simulink model "sl_subsys_fcncallerr10"  (Simulink 7.6)
settings: Solver=FixedStepDiscrete  StartTime=0.0  StopTime=10.0  FixedStep=1  RelTol=1e-3
Description:
  | Nested data dependency violation
  | 
  | To execute f2() we require that its data input, d be
  | valid. This means f1/Gain must execute before f1/chart2.
  | However, f1/chart2 is driving f1/Gain resulting in
  | a data dependency violation.
settings Model: Creator=The MathWorks Inc.  CovMetricSettings=d  ExtModeAutoUpdateStatusClock=off
settings OptimizationCC: BlockReduction=off  BooleanDataType=off  InlineInvariantSignals=on  InitFltsAndDblsToZero=on
settings DebuggingCC: SaveWithParameterizedLinksMsg=none  SignalResolutionControl=TryResolveAllWithWarning  SolverPrmCheckMsg=none  MultiTaskDSMMsg=warning  MultiTaskCondExecSysMsg=none  UnconnectedInputMsg=none  UnconnectedOutputMsg=none  UnconnectedLineMsg=none
settings HardwareCC: TargetUnknown=on
settings SFSimCC: SimParseCustomCode=off
settings RTWCC: IncludeERTFirstTime=on
settings CodeAppCC: CustomSymbolStrFcn=$F$N$M
settings GRTTargetCC: TargetFcnLib=ansi_tfl_tmw.mat

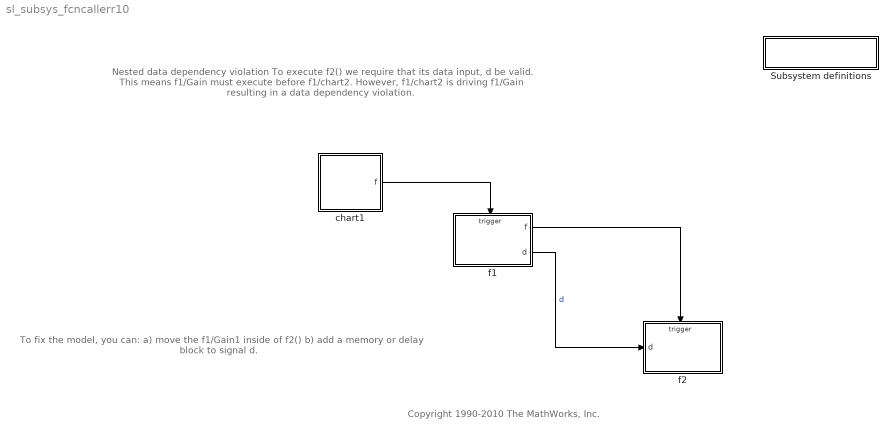
== system sl_subsys_fcncallerr10 ==
  note: Nested data dependency violation
      |
      | To execute f2() we require that its data input, d be
      | valid. This means f1/Gain must execute before f1/chart2.
      | However, f1/chart2 is driving f1/Gain resulting in
      | a data dependency violation.
  note: To fix the model, you can:
      | a)  move the f1/Gain1 inside of f2()
      | b) add a memory or delay block to signal d.
  note: Copyright 1990-2010 The MathWorks, Inc.
  " Subsystem definitions" : Subsystem
      settings: OpenFcn=helpview([matlabroot,'/toolbox/simulink/simdemos/simfeatures/html/sl_subsys_definitions.html']);
      mask Display: disp('Subsystem\ndefinitions')
  chart1 : Stateflow chart  TreatAsAtomicUnit=on
  f1 : Subsystem  TreatAsAtomicUnit=on
  f2 : Subsystem  TreatAsAtomicUnit=on
  wires:
  chart1/1(f) -> f1/Trigger
  f1/1(f) -> f2/Trigger
  f1/2(d) -> f2/1(d)  "d"

== system sl_subsys_fcncallerr10/ Subsystem definitions ==

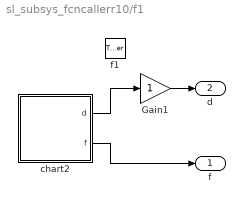
== system sl_subsys_fcncallerr10/f1 ==
  f1 : TriggerPort  TriggerType=function-call
  Gain1 : Gain  SaturateOnIntegerOverflow=on  OutDataTypeStr=Inherit: Same as input  ParamDataTypeStr=Inherit: Same as input
  chart2 : Stateflow chart  TreatAsAtomicUnit=on
  f : Outport
  d : Outport  Port=2
  wires:
  chart2/1(d) -> Gain1/1
  chart2/2(f) -> f/1
  Gain1/1 -> d/1

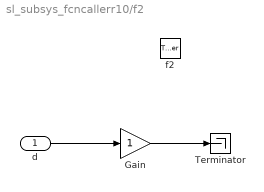
== system sl_subsys_fcncallerr10/f2 ==
  d : Inport
  f2 : TriggerPort  TriggerType=function-call
  Gain : Gain  SaturateOnIntegerOverflow=on  OutDataTypeStr=Inherit: Same as input  ParamDataTypeStr=Inherit: Same as input
  Terminator : Terminator
  wires:
  d/1 -> Gain/1
  Gain/1 -> Terminator/1

== stateflow chart chart1 ==
  state one/
    entry: f;
  state two/
    entry: f;
  one -> two
  two -> one
  (default) -> one
  events: f output FUNCTION_CALL_EVENT

== stateflow chart f1/chart2 ==
  state one/
    entry: f; d=1;
  state two/
    entry: f; d=2;
  one -> two
  two -> one
  (default) -> one
  data: d output double
  events: f output FUNCTION_CALL_EVENT
